simulink model "PID_subsystem"  (R2020b)
settings: Solver=VariableStepAuto  StartTime=0.0  StopTime=10.0  RelTol=1e-3
settings Model: Creator=Shivashis  LastModifiedBy=Shivashis
settings DataIOCC: SaveOutput=off  SaveTime=off

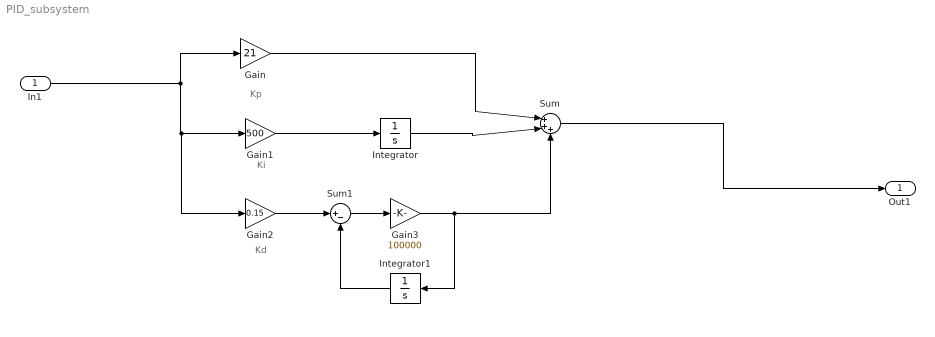
== system PID_subsystem ==
  note: Kd
  note: Ki
  note: Kp
  In1 : Inport  OutDataTypeStr=double  PortDimensions=1  SampleTime=0
  Gain : Gain  Gain=21
  Gain1 : Gain  Gain=500
  Gain2 : Gain  Gain=0.15
  Gain3 : Gain  Gain=100000
  Integrator : Integrator
  Integrator1 : Integrator
  Sum : Sum  Inputs=|+++
  Sum1 : Sum  Inputs=|+-
  Out1 : Outport  OutDataTypeStr=double  PortDimensions=1  SampleTime=0
  wires:
  Integrator/1 -> Sum/2
  In1/1 -> Gain2/1, Gain1/1, Gain/1
  Integrator1/1 -> Sum1/2
  Gain/1 -> Sum/1
  Sum1/1 -> Gain3/1
  Sum/1 -> Out1/1
  Gain1/1 -> Integrator/1
  Gain3/1 -> Sum/3, Integrator1/1
  Gain2/1 -> Sum1/1
